simulink model "Flowchart10"  (Simulink 8.7)
settings: Solver=FixedStepDiscrete  StartTime=0.0  StopTime=10.0  RelTol=1e-3
settings Model: Creator=scaife  LastModifiedBy=bourbouh  ExtModeAutoUpdateStatusClock=off
settings DataIOCC: SignalLoggingSaveFormat=ModelDataLogs  SignalLoggingName=sigsOut
settings OptimizationCC: InitFltsAndDblsToZero=on
settings DebuggingCC: SaveWithParameterizedLinksMsg=none  SignalResolutionControl=TryResolveAllWithWarning  MultiTaskDSMMsg=warning  MultiTaskCondExecSysMsg=none  StrictBusMsg=None
settings HardwareCC: TargetUnknown=on
settings SFSimCC: SimParseCustomCode=off
settings GRTTargetCC: TargetFcnLib=ansi_tfl_tmw.mat  ModelReferenceCompliant=off  ParMdlRefBuildCompliant=off  CompOptLevelCompliant=off  ConcurrentExecutionCompliant=off  GeneratePreprocessorConditionals=Use local settings  CombineOutputUpdateFcns=off  MatFileLogging=off  MATLABClassNameForMDSCustomization=Simulink.SoftwareTarget.TargetSpecificTriggerConfigurationBase  GRTInterface=on

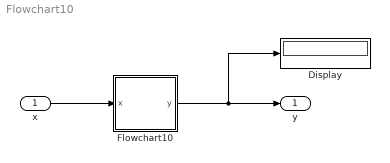
== system Flowchart10 ==
  x : Inport
  Display : Display
  Flowchart10 : Stateflow chart  TreatAsAtomicUnit=on
  y : Outport
  wires:
  Flowchart10/1(y) -> y/1, Display/1
  x/1 -> Flowchart10/1(x)

== stateflow chart Flowchart10 ==
  state A [parallel]
    settings: executionOrder=1
    (default) -> (junction 4) [order 1] : [x==0]{y++;}
    (default) -> (junction 5) [order 2] : [x>0]{y--;}
    A -> (junction 6) [order 2] : [x==0]{y+=2;}
    A -> (junction 7) [order 1] : [x>0]{y-=2;}
  data: x input int32; y output int32
